simulink model "mech_user_added_css"  (R2017b)
settings: Solver=ode45  StartTime=0.0  StopTime=10.0  MaxStep=0.2  RelTol=1e-3  EnableMultiTasking=on
undefined symbols (not defined in the file): Base, gear1, gear2, GearAssembly, RootGround, RootPart
libraries: mblibv1 x12
Description:
  | User-Added Coordinate Systems in an Imported Gear Assembly
  | 
  | This example shows the user added coordinate systems imported from a CAD assembly.
  | 
  | Copyright 2009-2017 The MathWorks, Inc.
settings Model: Creator=MathWorks  LastModifiedBy=smiller
settings DataIOCC: LimitDataPoints=on  SaveFormat=Array  SignalLoggingSaveFormat=ModelDataLogs
settings OptimizationCC: ExpressionDepthLimit=2147483647  LifeSpan=inf
settings DebuggingCC: UnderspecifiedInitializationDetection=Classic  MergeDetectMultiDrivingBlocksExec=none  SolverPrmCheckMsg=warning  FcnCallInpInsideContextMsg=warning  StateNameClashWarn=warning  SFUnexpectedBacktrackingDiag=warning  SFNoUnconditionalDefaultTransitionDiag=warning  SFExecutionAtInitializationDiag=none
settings HardwareCC: ProdBitPerPointer=32  ProdBitPerSizeT=32  ProdBitPerPtrDiffT=32  ProdLargestAtomicFloat=None  ProdIntDivRoundTo=Undefined  ProdEndianess=Unspecified  ProdWordSize=32  ProdHWDeviceType=32-bit Generic
settings ModelReferenceCC: PropagateSignalLabelsOutOfModel=off
settings CodeAppCC: StateflowObjectComments=on
settings GRTTargetCC: TargetLangStandard=C89/C90 (ANSI)  GeneratePreprocessorConditionals=Disable all  CombineOutputUpdateFcns=off  GRTInterface=on
settings ConfigComp: CovMetricSettings=dw  CovHtmlReporting=on  CovSaveCumulativeToWorkspaceVar=on  CovSaveSingleToWorkspaceVar=on  CovExternalEMLEnable=off
settings SimscapeCC: SimscapeNormalizeSystem=off
settings SimMechanicsCC: VisOnUpdateDiagram=on  VisDuringSimulation=on  LastVizWinPosition=[680 678 560 420]  CamPosition=[6.49573;6.50956;6.5455;]  CamTarget=[-0.0127727;0.00105815;0.037;]  CamUpVector=[0;1;0;]  CamHeight=0.285099  VisBackgroundColor=[0.9;0.9;0.95;]  DefaultBodyColor=[1;0;0;]
settings ConfigurationSet: Description=SimMechanics 2G

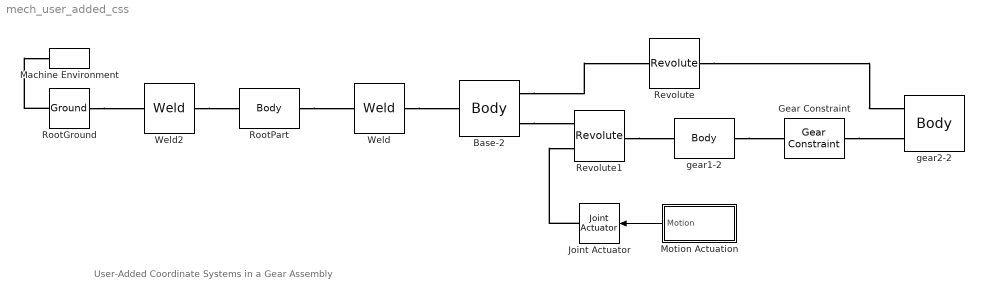
== system mech_user_added_css ==
  note: User-Added Coordinate Systems in a Gear Assembly
  Base-2 : mblibv1/Bodies/Body  LConnTagsString=CS2  RConnTagsString=CS3|CS4  UpdateFromCAD=on  PMImportedID=Base-2  DialogClass=MechanicalBodyBlock  Mass=0.30604  MassUnits=kg  InertiaUnits=kg*m^2  Inertia=[0.000565844,0,1.57386e-006;0,0.00101417,0;1.57386e-006,0,0.00157373]  Shape=Cylinder  ShapeDims=[1 1]  ShapeUnits=m  ShapeUse=false  Density=1  DensityUnits=kg/m^3  DensityUse=false  GraphicsMode=GFXFILE  GraphicsFileName=GearAssembly-Base-2.STL  BodyColorSelMode=COLORPALETTE  BodyColor=[0.75294 0.75294 0.75294]  AttachedToCS=CS1  CG=Right$CG$[-0.00479576 0.000958827 0.00519735]$WORLD$WORLD$m$[1 0 0;0 1 0;0 0 1]$3x3 Transform$rad$WORLD$false$Base-2::CG(AUTOGEN)  WorkingFrames=Right$CS1$[0.0236501 0.0322309 0]$WORLD$WORLD$m$[1 0 0;0 1 0;0 0 1]$3x3 Transform$rad$WORLD$false$Base-2::CS1(AUTOGEN)#Left$CS2$[-0.00479576 0.000958827 0.00519735]$WORLD$WORLD$m$[1 0 0;0 1 0;0 0 1]$3x3 Transform$rad$WORLD$true$Base-2:-:GearAssembly/RootPart::Base-2(AUTOGEN)#Right$CS3$[0.0382289 0.000958827 0.02]$WORLD$WORLD$m$[1 0 0;0 1 0;0 0 1]$3x3 Transform$rad$WORLD$true$Base-2:-:gear2-2::Base-2(AUTOGEN)#Right$CS4$[-0.0467711 0.000958827 0.02]$WORLD$WORLD$m$[1 0 0;0 1 0;0 0 1]$3x3 Transform$rad$WORLD$true$Base-2:-:gear1-2::Base-2(AUTOGEN)  CGPos=[-0.00479576 0.000958827 0.00519735]  CGRot=[1 0 0;0 1 0;0 0 1]  CS0Pos=[]  CS0Rot=[]  CS1Pos=[0.0236501 0.0322309 0]  CS1Rot=[1 0 0;0 1 0;0 0 1]  CS2Pos=[-0.00479576 0.000958827 0.00519735]  CS2Rot=[1 0 0;0 1 0;0 0 1]  CS3Pos=[0.0382289 0.000958827 0.02]  CS3Rot=[1 0 0;0 1 0;0 0 1]  CS4Pos=[-0.0467711 0.000958827 0.02]  CS4Rot=[1 0 0;0 1 0;0 0 1]  CS5Pos=[]  CS5Rot=[]  CS6Pos=[]  CS6Rot=[]  CS7Pos=[]  CS7Rot=[]  CS8Pos=[]  CS8Rot=[]  CS9Pos=[]  CS9Rot=[]  CS10Pos=[]  CS10Rot=[]  CS11Pos=[]  CS11Rot=[]  CS12Pos=[]  CS12Rot=[]  CS13Pos=[]  CS13Rot=[]  CS14Pos=[]  CS14Rot=[]  CS15Pos=[]  CS15Rot=[]  CS16Pos=[]  CS16Rot=[]  CS17Pos=[]  CS17Rot=[]  CS18Pos=[]  CS18Rot=[]  CS19Pos=[]  CS19Rot=[]  CS20Pos=[]  CS20Rot=[]
      settings: SourceProductName=Simscape Multibody  SourceProductBaseCode=MS
  Gear Constraint : mblibv1/Constraints &  Drivers/Gear Constraint  LConnTagsString=__newl0  RConnTagsString=__newr0  UpdateFromCAD=off  DialogClass=GearConstraint  NumSAPorts=0  BaseRadius=50  BaseRadiusUnits=mm  FollowerRadius=35  FollowerRadiusUnits=mm
      settings: SourceProductName=Simscape Multibody  SourceProductBaseCode=MS
  Joint Actuator : mblibv1/Sensors &  Actuators/Joint Actuator  UpdateFromCAD=off  PhysicalDomain=Mechanical  PortType=blob  ActuationStyle=Motion  AngleUnits=rad  ArcVelocityUnits=rad/s  ArcAccelerationUnits=rad/s^2  CoordPositionUnits=m  VelocityUnits=m/s  AccelerationUnits=m/s^2  ForceUnits=N  TorqueUnits=N-m  ActiveIO=on  Width=3  DialogClass=MechanicalActuatorBlock  Primitive=R1  ReferenceFrame=Absolute (INERTIAL)
      settings: SourceProductName=Simscape Multibody  SourceProductBaseCode=MS
  Machine Environment : mblibv1/Bodies/Machine Environment  PortType=env  PhysicalDomain=Mechanical  DialogTemplateClass=MECH.MachineEnvironment  SyncWhenCopied=off  Gravity=[0 -9.81 0]  GravityUnits=m/s^2  GravityAsSignal=off  Dimensionality=Auto-detect  AnalysisType=Forward dynamics  LinearAssemblyTolerance=1e-3  LinearAssemblyToleranceUnits=m  AngularAssemblyTolerance=1e-3  AngularAssemblyToleranceUnits=rad  ConstraintSolverType=Stabilizing  ConstraintRelTolerance=1e-4  ConstraintAbsTolerance=1e-4  UseRobustSingularityHandling=off  RedundancyAnalysisToleranceType=Automatically select tolerance  RedundancyAnalysisTolerance=1e-14  StatePerturbationType=Fixed  PerturbationSize=1e-5  VisualizeMachine=on  BodyVisualizationType=Use model default body geometries  BodyColorSelMode=Use model default  DefaultBodyColor=[1 0 0]
      settings: SourceProductName=Simscape Multibody  SourceProductBaseCode=MS
  Motion Actuation : Subsystem
  Revolute : mblibv1/Joints/Revolute  LConnTagsString=__newl0  RConnTagsString=__newr0  UpdateFromCAD=on  PMImportedID=Base-2:-:gear2-2  NumSAPorts=0  CutJoint=off  MarkAsCut=off  Primitives=prismatic  PrimitiveProps=R1$WORLD$[0,0,-1]$revolute  DialogClass=JointBlock  R1Axis=[0,0,-1]
      settings: SourceProductName=Simscape Multibody  SourceProductBaseCode=MS
  Revolute1 : mblibv1/Joints/Revolute  LConnTagsString=__newl0|SA1  RConnTagsString=__newr0  UpdateFromCAD=on  PMImportedID=Base-2:-:gear1-2  NumSAPorts=1  CutJoint=off  MarkAsCut=off  Primitives=prismatic  PrimitiveProps=R1$World$[0,0,-1]$revolute  DialogClass=JointBlock  R1Axis=[0,0,-1]
      settings: SourceProductName=Simscape Multibody  SourceProductBaseCode=MS
  RootGround : mblibv1/Bodies/Ground  UpdateFromCAD=on  PMImportedID=RootGround  LeftPortType=env  RightPortType=workingframe  PhysicalDomain=Mechanical  DialogClass=GroundBlock  CoordPosition=[-0.0127472,0.000958827,0.0149261]  CoordPositionUnits=m  StateVectorMgrId=-1  MachineId=[0 0]  ShowEnvPort=on  ParameterChecksum=[0 0 0 0]  TopologyChecksum=[0 0 0 0]
      settings: SourceProductName=Simscape Multibody  SourceProductBaseCode=MS
  RootPart : mblibv1/Bodies/Body  LConnTagsString=CS3  RConnTagsString=CS2  UpdateFromCAD=on  PMImportedID=GearAssembly/RootPart  DialogClass=MechanicalBodyBlock  Mass=0  MassUnits=kg  InertiaUnits=kg*m^2  Inertia=[0,0,0;0,0,0;0,0,0]  Shape=Cylinder  ShapeDims=[1 1]  ShapeUnits=m  ShapeUse=false  Density=1  DensityUnits=kg/m^3  DensityUse=false  GraphicsMode=MACHINE_DEFAULT  BodyColorSelMode=MACHINE_DEFAULT  BodyColor=[1 0 0]  AttachedToCS=CS1  CG=Right$CG$[-0.0127472 0.000958827 0.0149261]$WORLD$WORLD$m$[1 0 0;0 1 0;0 0 1]$3x3 Transform$rad$WORLD$false$GearAssembly/RootPart::CG(AUTOGEN)  WorkingFrames=Right$CS1$[0 0 0]$WORLD$WORLD$m$[1 0 0;0 1 0;0 0 1]$3x3 Transform$rad$WORLD$false$GearAssembly/RootPart::CS1(AUTOGEN)#Right$CS2$[-0.00479576 0.000958827 0.00519735]$WORLD$WORLD$m$[1 0 0;0 1 0;0 0 1]$3x3 Transform$rad$WORLD$true$Base-2:-:GearAssembly/RootPart::GearAssembly/RootPart(AUTOGEN)#Left$CS3$[-0.0127472 0.000958827 0.0149261]$WORLD$WORLD$m$[1 0 0;0 1 0;0 0 1]$3x3 Transform$rad$WORLD$true$GearAssembly/RootPart:-:RootGround::GearAssembly/RootPart(AUTOGEN)  CGPos=[-0.0127472 0.000958827 0.0149261]  CGRot=[1 0 0;0 1 0;0 0 1]  CS0Pos=[]  CS0Rot=[]  CS1Pos=[0 0 0]  CS1Rot=[1 0 0;0 1 0;0 0 1]  CS2Pos=[-0.00479576 0.000958827 0.00519735]  CS2Rot=[1 0 0;0 1 0;0 0 1]  CS3Pos=[-0.0127472 0.000958827 0.0149261]  CS3Rot=[1 0 0;0 1 0;0 0 1]  CS4Pos=[]  CS4Rot=[]  CS5Pos=[]  CS5Rot=[]  CS6Pos=[]  CS6Rot=[]  CS7Pos=[]  CS7Rot=[]  CS8Pos=[]  CS8Rot=[]  CS9Pos=[]  CS9Rot=[]  CS10Pos=[]  CS10Rot=[]  CS11Pos=[]  CS11Rot=[]  CS12Pos=[]  CS12Rot=[]  CS13Pos=[]  CS13Rot=[]  CS14Pos=[]  CS14Rot=[]  CS15Pos=[]  CS15Rot=[]  CS16Pos=[]  CS16Rot=[]  CS17Pos=[]  CS17Rot=[]  CS18Pos=[]  CS18Rot=[]  CS19Pos=[]  CS19Rot=[]  CS20Pos=[]  CS20Rot=[]
      settings: SourceProductName=Simscape Multibody  SourceProductBaseCode=MS
  Weld : mblibv1/Joints/Weld  LConnTagsString=__newl0  RConnTagsString=__newr0  UpdateFromCAD=on  PMImportedID=Base-2:-:GearAssembly/RootPart  NumSAPorts=0  CutJoint=off  MarkAsCut=off  Primitives=weld  PrimitiveProps=W$WORLD$[0.57735,0.57735,0.57735]$weld  DialogClass=JointBlock  WAxis=[0.57735,0.57735,0.57735]
      settings: SourceProductName=Simscape Multibody  SourceProductBaseCode=MS
  Weld2 : mblibv1/Joints/Weld  LConnTagsString=__newl0  RConnTagsString=__newr0  UpdateFromCAD=on  PMImportedID=GearAssembly/RootPart:-:RootGround  NumSAPorts=0  CutJoint=off  MarkAsCut=off  Primitives=weld  PrimitiveProps=W$WORLD$[0.57735,0.57735,0.57735]$weld  DialogClass=JointBlock  WAxis=[0.57735,0.57735,0.57735]
      settings: SourceProductName=Simscape Multibody  SourceProductBaseCode=MS
  gear1-2 : mblibv1/Bodies/Body  LConnTagsString=CS4  RConnTagsString=CS2  UpdateFromCAD=on  PMImportedID=gear1-2  DialogClass=MechanicalBodyBlock  Mass=0.113676  MassUnits=kg  InertiaUnits=kg*m^2  Inertia=[8.65316e-005,-2.11247e-005,-1.38594e-005;-2.11247e-005,0.000114269,2.56782e-005;-1.38594e-005,2.56782e-005,9.19768e-005]  Shape=Cylinder  ShapeDims=[1 1]  ShapeUnits=m  ShapeUse=false  Density=1  DensityUnits=kg/m^3  DensityUse=false  GraphicsMode=GFXFILE  GraphicsFileName=GearAssembly-gear1-2.STL  BodyColorSelMode=COLORPALETTE  BodyColor=[0.75294 0.75294 1]  AttachedToCS=CS1  CG=Right$CG$[-0.0467711 0.000958827 0.035927]$WORLD$WORLD$m$[-0.220543 -0.615471 0.756674;-0.884401 -0.200974 -0.421241;0.411334 -0.762105 -0.5]$3x3 Transform$rad$WORLD$false$gear1-2::CG(AUTOGEN)  WorkingFrames=Right$CS1$[-0.0467711 0.000958827 0.0750448]$WORLD$WORLD$m$[-0.220543 -0.615471 0.756674;-0.884401 -0.200974 -0.421241;0.411334 -0.762105 -0.5]$3x3 Transform$rad$WORLD$false$gear1-2::CS1(AUTOGEN)#Right$CS2$[-0.0467711 0.000958827 0.032]$WORLD$WORLD$m$[-0.24196 0 -0.970286;-0.970286 0 0.24196;0 1 0]$3x3 Transform$rad$WORLD$true$SMLINK_CS1(USERADDED)#Right$CS3$[-0.0467711 0.000958827 0.035927]$WORLD$WORLD$m$[1 0 0;0 1 0;0 0 1]$3x3 Transform$rad$WORLD$false$gear1-2:-:gear2-2::gear1-2(AUTOGEN)#Left$CS4$[-0.0467711 0.000958827 0.02]$WORLD$WORLD$m$[1 0 0;0 1 0;0 0 1]$3x3 Transform$rad$WORLD$true$Base-2:-:gear1-2::gear1-2(AUTOGEN)  CGPos=[-0.0467711 0.000958827 0.035927]  CGRot=[-0.220543 -0.615471 0.756674;-0.884401 -0.200974 -0.421241;0.411334 -0.762105 -0.5]  CS0Pos=[]  CS0Rot=[]  CS1Pos=[-0.0467711 0.000958827 0.0750448]  CS1Rot=[-0.220543 -0.615471 0.756674;-0.884401 -0.200974 -0.421241;0.411334 -0.762105 -0.5]  CS2Pos=[-0.0467711 0.000958827 0.032]  CS2Rot=[-0.24196 0 -0.970286;-0.970286 0 0.24196;0 1 0]  CS3Pos=[-0.0467711 0.000958827 0.035927]  CS3Rot=[1 0 0;0 1 0;0 0 1]  CS4Pos=[-0.0467711 0.000958827 0.02]  CS4Rot=[1 0 0;0 1 0;0 0 1]  CS5Pos=[]  CS5Rot=[]  CS6Pos=[]  CS6Rot=[]  CS7Pos=[]  CS7Rot=[]  CS8Pos=[]  CS8Rot=[]  CS9Pos=[]  CS9Rot=[]  CS10Pos=[]  CS10Rot=[]  CS11Pos=[]  CS11Rot=[]  CS12Pos=[]  CS12Rot=[]  CS13Pos=[]  CS13Rot=[]  CS14Pos=[]  CS14Rot=[]  CS15Pos=[]  CS15Rot=[]  CS16Pos=[]  CS16Rot=[]  CS17Pos=[]  CS17Rot=[]  CS18Pos=[]  CS18Rot=[]  CS19Pos=[]  CS19Rot=[]  CS20Pos=[]  CS20Rot=[]
      settings: SourceProductName=Simscape Multibody  SourceProductBaseCode=MS
  gear2-2 : mblibv1/Bodies/Body  LConnTagsString=CS4|CS2  UpdateFromCAD=on  PMImportedID=gear2-2  DialogClass=MechanicalBodyBlock  Mass=0.0281355  MassUnits=kg  InertiaUnits=kg*m^2  Inertia=[5.26803e-006,0,0;0,5.26803e-006,0;0,0,8.56695e-006]  Shape=Cylinder  ShapeDims=[1 1]  ShapeUnits=m  ShapeUse=false  Density=1  DensityUnits=kg/m^3  DensityUse=false  GraphicsMode=GFXFILE  GraphicsFileName=GearAssembly-gear2-2.STL  BodyColorSelMode=COLORPALETTE  BodyColor=[0.75294 1 1]  AttachedToCS=CS1  CG=Right$CG$[0.0382289 0.000958827 0.0358984]$WORLD$WORLD$m$[0.559948 -0.828528 0;0.828528 0.559948 0;0 0 1]$3x3 Transform$rad$WORLD$false$gear2-2::CG(AUTOGEN)  WorkingFrames=Right$CS1$[0.0382289 0.000958827 0.032]$WORLD$WORLD$m$[0.559948 -0.828528 0;0.828528 0.559948 0;0 0 1]$3x3 Transform$rad$WORLD$false$gear2-2::CS1(AUTOGEN)#Left$CS4$[0.0382289 0.000958827 0.02]$WORLD$WORLD$m$[1 0 0;0 1 0;0 0 1]$3x3 Transform$rad$WORLD$true$Base-2:-:gear2-2::gear2-2(AUTOGEN)#Left$CS2$[0.0382289 0.000958827 0.032]$WORLD$WORLD$m$[0.559948 -0.828528 0;0.828528 0.559948 0;0 0 1]$3x3 Transform$rad$WORLD$true$SMLINK_CS2(USERADDED)#Left$CS3$[-0.0467711 0.000958827 0.035927]$WORLD$WORLD$m$[1 0 0;0 1 0;0 0 1]$3x3 Transform$rad$WORLD$false$gear1-2:-:gear2-2::gear2-2(AUTOGEN)  CGPos=[0.0382289 0.000958827 0.0358984]  CGRot=[0.559948 -0.828528 0;0.828528 0.559948 0;0 0 1]  CS0Pos=[]  CS0Rot=[]  CS1Pos=[0.0382289 0.000958827 0.032]  CS1Rot=[0.559948 -0.828528 0;0.828528 0.559948 0;0 0 1]  CS2Pos=[0.0382289 0.000958827 0.032]  CS2Rot=[0.559948 -0.828528 0;0.828528 0.559948 0;0 0 1]  CS3Pos=[-0.0467711 0.000958827 0.035927]  CS3Rot=[1 0 0;0 1 0;0 0 1]  CS4Pos=[0.0382289 0.000958827 0.02]  CS4Rot=[1 0 0;0 1 0;0 0 1]  CS5Pos=[]  CS5Rot=[]  CS6Pos=[]  CS6Rot=[]  CS7Pos=[]  CS7Rot=[]  CS8Pos=[]  CS8Rot=[]  CS9Pos=[]  CS9Rot=[]  CS10Pos=[]  CS10Rot=[]  CS11Pos=[]  CS11Rot=[]  CS12Pos=[]  CS12Rot=[]  CS13Pos=[]  CS13Rot=[]  CS14Pos=[]  CS14Rot=[]  CS15Pos=[]  CS15Rot=[]  CS16Pos=[]  CS16Rot=[]  CS17Pos=[]  CS17Rot=[]  CS18Pos=[]  CS18Rot=[]  CS19Pos=[]  CS19Rot=[]  CS20Pos=[]  CS20Rot=[]
      settings: SourceProductName=Simscape Multibody  SourceProductBaseCode=MS
  wires:
  Motion Actuation/1(Motion) -> Joint Actuator/1
  connections:
  RootPart/RConn1 -- Weld/LConn1
  Weld/RConn1 -- Base-2/LConn1
  Revolute/RConn1 -- gear2-2/LConn1
  Base-2/RConn2 -- Revolute1/LConn1
  Revolute1/RConn1 -- gear1-2/LConn1
  RootGround/RConn1 -- Weld2/LConn1
  Weld2/RConn1 -- RootPart/LConn1
  RootGround/LConn1 -- Machine Environment/RConn1
  gear1-2/RConn1 -- Gear Constraint/LConn1
  Gear Constraint/RConn1 -- gear2-2/LConn2
  Joint Actuator/RConn1 -- Revolute1/LConn2
  Base-2/RConn1 -- Revolute/LConn1

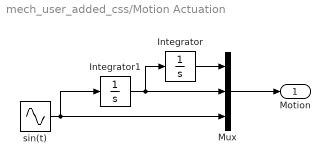
== system mech_user_added_css/Motion Actuation ==
  Integrator : Integrator
  Integrator1 : Integrator  InitialCondition=-0.25
  Mux : Mux  Inputs=3
  sin(t) : Sin  Amplitude=0.5  SampleTime=0
  Motion : Outport
  wires:
  Mux/1 -> Motion/1
  Integrator1/1 -> Mux/2, Integrator/1
  sin(t)/1 -> Mux/3, Integrator1/1
  Integrator/1 -> Mux/1
